simulink model "QSS_HEV"  (R2024a)
settings: Solver=VariableStepDiscrete  StartTime=0.0  StopTime=1220  RelTol=1e-3  EnableMultiTasking=on
undefined symbols (not defined in the file or in its folder): eta_EM_map, h, H_u, P_MGB_FTP75, PMGB_NEDC, rho_f, T_CE_max, T_EM_max, V_CE_map, w_CE_max, w_EM_row
libraries: qss_tb_library x7, simulink x2, dspindex x2, mpclib x1
settings Model: Creator=d_goerges  LastModifiedBy=apple
settings SolverCC: AlgebraicLoopSolver=TrustRegion
settings DataIOCC: LimitDataPoints=on  SaveFormat=Array  SignalLoggingSaveFormat=ModelDataLogs  ReturnWorkspaceOutputs=off
settings OptimizationCC: ExpressionDepthLimit=2147483647  LifeSpan=inf
settings DebuggingCC: UnderspecifiedInitializationDetection=Classic  MergeDetectMultiDrivingBlocksExec=none  SolverPrmCheckMsg=warning  FcnCallInpInsideContextMsg=warning  UnconnectedInputMsg=warning  UnconnectedOutputMsg=warning  UnconnectedLineMsg=warning  StateNameClashWarn=warning  SFUnexpectedBacktrackingDiag=warning  SFNoUnconditionalDefaultTransitionDiag=warning  SFExecutionAtInitializationDiag=none  ArithmeticOperatorsInVariantConditions=warning
settings HardwareCC: ProdBitPerPointer=32  ProdBitPerSizeT=32  ProdBitPerPtrDiffT=32  ProdLargestAtomicFloat=None  ProdIntDivRoundTo=Undefined  ProdEndianess=Unspecified  ProdWordSize=32  ProdHWDeviceType=32-bit Generic
settings ModelReferenceCC: PropagateSignalLabelsOutOfModel=off
settings SFSimCC: SimUseLocalCustomCode=off  CustomCodeUndefinedFunction=UseInterfaceOnly
settings RTWCC: RTWUseLocalCustomCode=off  GPUComputeCapability=3.5
settings CodeAppCC: StateflowObjectComments=on
settings GRTTargetCC: TargetLangStandard=C89/C90 (ANSI)  CombineOutputUpdateFcns=off  GRTInterface=on
settings ConfigComp: CovMetricSettings=dw  CovSaveCumulativeToWorkspaceVar=on  CovSaveSingleToWorkspaceVar=on  CovExternalEMLEnable=off

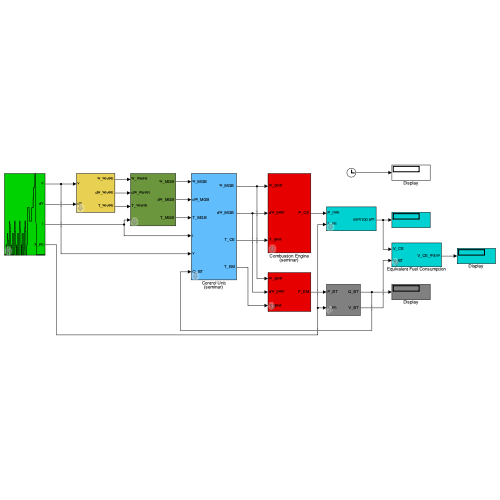
[thumbnail: Simulink's stored preview of the top-level diagram]
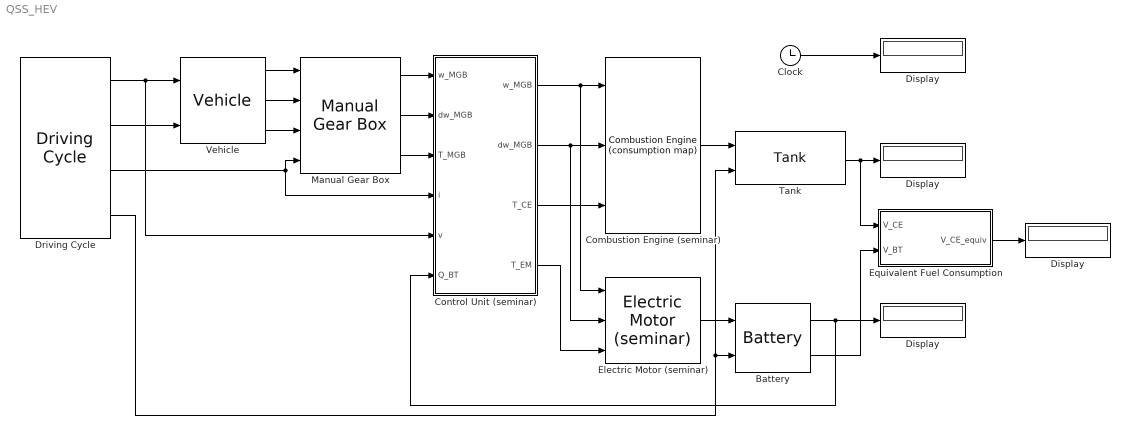
== system QSS_HEV ==
  "   Display   " : Display
  "  Display  " : Display
  " Display " : Display
  Battery : qss_tb_library/Energy Buffer/Battery  Tag=battery  I_0=10  Q_BT_IC_rel=50  t_ch=2
  Clock : Clock
  Combustion Engine (seminar) : qss_tb_library/Energy Converter/Combustion Engine (consumption map)  Tag=combustion engine  theta_CE=0.2  w_CE_idle=105  P_CE_idle=8000  P_aux=0  ENABLE_FUEL_CUTOFF=on  T_CE_cutoff=5  P_CE_cutoff=0
  Control Unit (seminar) : Subsystem  Tag=control unit  mask(Control Unit){}
      mask help:
      | This block gives the user the opportunity to design his/her own control unit.
      |
      | The user can define the inputs and outputs  by himself/herself.
      mask init:
      | %init_control_unit;
  Display : Display
  Driving Cycle : qss_tb_library/Driving Cycle/Driving Cycle  Tag=cycle  cyclenr=Europe: NEDC  stepsize=1  autostop=on
  Electric Motor (seminar) : qss_tb_library/Energy Converter/Electric Motor (seminar)  theta_EM=0.1  P_aux=0
  Equivalent Fuel Consumption : Subsystem  mask(Equivalent Fuel Consumption){eta_BT=0.9, eta_EM=0.8, eta_CE=0.25}
      mask prompts: eta_BT "Battery efficiency [-]"; eta_EM "Motor efficiency [-]"; eta_CE "Engine efficiency [-]"
      mask help:
      | This block computes the equivalent fuel consumption.
      |
      | Input:
      | =====
      | 	V_CE    Fuel consumption [l/100 km]
      | 	V_BT    Energy consumption [kWh/100 km]
      |
      | Output:
      | ======
      | 	V_CE_equiv	Equivalent fuel consumption [l/100 km]
      mask init:
      | init_equivalent_fuel_consumption;
  Manual Gear Box : qss_tb_library/Gear System/Manual Gear Box  Tag=transmission  i_1=3.27  i_2=1.92  i_3=1.26  i_4=0.88  i_5=0.7  i_diff=3.29  e_GT=0.98  P_GT0=100  w_wheel_min=1
  Tank : qss_tb_library/Energy Source/Tank  Tag=tank  fuel=Diesel  flag_cold_start=on
  Vehicle : qss_tb_library/Vehicle/Vehicle  Tag=vehicle  m_f=1115  mt2m_f=5  A_f=2.3  d_wheel=0.576  cw=0.31  mu=0.013
  wires:
  Tank/1 -> Display/1, Equivalent Fuel Consumption/1(V_CE)
  Driving Cycle/2 -> Vehicle/2
  Driving Cycle/1 -> Vehicle/1, Control Unit (seminar)/5(v)
  Vehicle/1 -> Manual Gear Box/1
  Vehicle/2 -> Manual Gear Box/2
  Vehicle/3 -> Manual Gear Box/3
  Manual Gear Box/1 -> Control Unit (seminar)/1(w_MGB)
  Manual Gear Box/2 -> Control Unit (seminar)/2(dw_MGB)
  Manual Gear Box/3 -> Control Unit (seminar)/3(T_MGB)
  Control Unit (seminar)/1(" w_MGB ") -> Combustion Engine (seminar)/1, Electric Motor (seminar)/1
  Control Unit (seminar)/2(" dw_MGB ") -> Combustion Engine (seminar)/2, Electric Motor (seminar)/2
  Control Unit (seminar)/3(T_CE) -> Combustion Engine (seminar)/3
  Control Unit (seminar)/4(T_EM) -> Electric Motor (seminar)/3
  Combustion Engine (seminar)/1 -> Tank/1
  Electric Motor (seminar)/1 -> Battery/1
  Driving Cycle/4 -> Battery/2, Tank/2
  Battery/1 -> "  Display  "/1, Control Unit (seminar)/6(Q_BT)
  Driving Cycle/3 -> Manual Gear Box/4, Control Unit (seminar)/4(i)
  Battery/2 -> Equivalent Fuel Consumption/2(V_BT)
  Clock/1 -> " Display "/1
  Equivalent Fuel Consumption/1(V_CE_equiv) -> "   Display   "/1

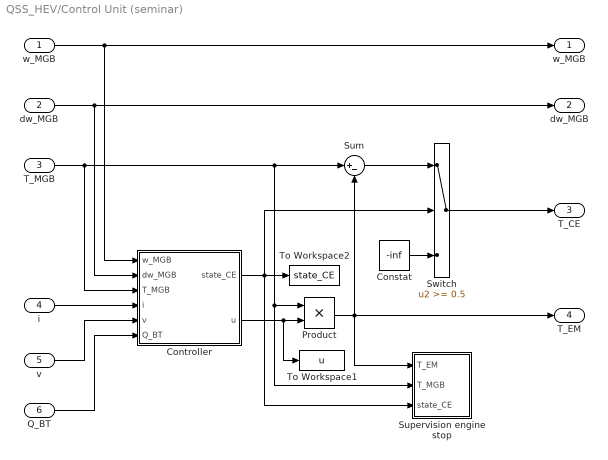
== system QSS_HEV/Control Unit (seminar) ==
  w_MGB : Inport
  dw_MGB : Inport  Port=2
  T_MGB : Inport  Port=3
  i : Inport  Port=4
  v : Inport  Port=5
  Q_BT : Inport  Port=6
  Constat : Constant  Value=-inf
  Controller : Subsystem  TreatAsAtomicUnit=on
  Product : Product  RndMeth=Zero
  Sum : Sum  Inputs=|+-
  Supervision engine stop : Subsystem
  Switch : Switch  Threshold=0.5  SaturateOnIntegerOverflow=off  InputSameDT=off
  To Workspace1 : ToWorkspace  VariableName=u  SampleTime=-1
  To Workspace2 : ToWorkspace  VariableName=state_CE  SampleTime=-1
  " w_MGB " : Outport  InitialOutput=0
  " dw_MGB " : Outport  Port=2  InitialOutput=0
  T_CE : Outport  Port=3  InitialOutput=0
  T_EM : Outport  Port=4  InitialOutput=0
  wires:
  dw_MGB/1 -> Controller/2(dw_MGB), " dw_MGB "/1
  w_MGB/1 -> Controller/1(w_MGB), " w_MGB "/1
  T_MGB/1 -> Controller/3(T_MGB), Sum/1, Product/1, Supervision engine stop/2(T_MGB)
  Product/1 -> Sum/2, T_EM/1, Supervision engine stop/1(T_EM)
  Controller/2(u) -> To Workspace1/1, Product/2
  i/1 -> Controller/4(i)
  Controller/1(state_CE) -> Switch/2, To Workspace2/1, Supervision engine stop/3(state_CE)
  Sum/1 -> Switch/1
  Switch/1 -> T_CE/1
  Constat/1 -> Switch/3
  v/1 -> Controller/5(v)
  Q_BT/1 -> Controller/6(Q_BT)

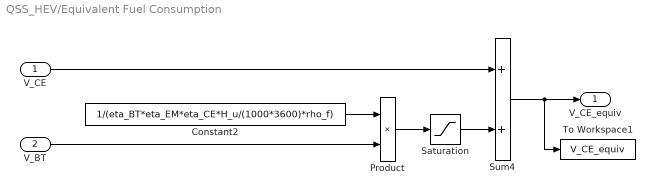
== system QSS_HEV/Equivalent Fuel Consumption ==
  V_CE : Inport
  V_BT : Inport  Port=2
  Constant2 : Constant  Value=1/(eta_BT*eta_EM*eta_CE*H_u/(1000*3600)*rho_f)
  Product : Product  RndMeth=Zero
  Saturation : Saturate  UpperLimit=inf  LowerLimit=0
  Sum4 : Sum  InputSameDT=on  SaturateOnIntegerOverflow=on  OutDataTypeStr=Inherit: Same as first input
  To Workspace1 : ToWorkspace  VariableName=V_CE_equiv  SampleTime=-1
  V_CE_equiv : Outport
  wires:
  Product/1 -> Saturation/1
  V_BT/1 -> Product/2
  Constant2/1 -> Product/1
  Sum4/1 -> To Workspace1/1, V_CE_equiv/1
  V_CE/1 -> Sum4/1
  Saturation/1 -> Sum4/2

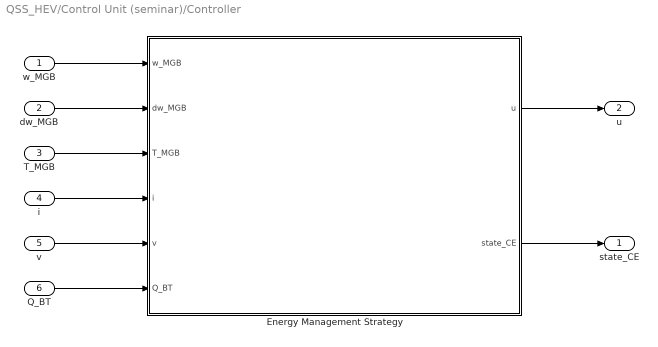
== system QSS_HEV/Control Unit (seminar)/Controller ==
  w_MGB : Inport
  dw_MGB : Inport  Port=2
  T_MGB : Inport  Port=3
  i : Inport  Port=4
  v : Inport  Port=5
  Q_BT : Inport  Port=6
  Energy Management Strategy : Subsystem
  state_CE : Outport  InitialOutput=0
  u : Outport  Port=2  InitialOutput=0
  wires:
  Energy Management Strategy/2(state_CE) -> state_CE/1
  Energy Management Strategy/1(u) -> u/1
  w_MGB/1 -> Energy Management Strategy/1(w_MGB)
  dw_MGB/1 -> Energy Management Strategy/2(dw_MGB)
  T_MGB/1 -> Energy Management Strategy/3(T_MGB)
  i/1 -> Energy Management Strategy/4(i)
  v/1 -> Energy Management Strategy/5(v)
  Q_BT/1 -> Energy Management Strategy/6(Q_BT)

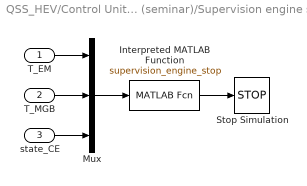
== system QSS_HEV/Control Unit (seminar)/Supervision engine stop ==
  T_EM : Inport
  T_MGB : Inport  Port=2
  state_CE : Inport  Port=3
  Interpreted MATLAB Function : MATLABFcn  MATLABFcn=supervision_engine_stop
  Mux : Mux  Inputs=3
  Stop Simulation : Stop
  wires:
  T_MGB/1 -> Mux/2
  T_EM/1 -> Mux/1
  state_CE/1 -> Mux/3
  Mux/1 -> Interpreted MATLAB Function/1
  Interpreted MATLAB Function/1 -> Stop Simulation/1

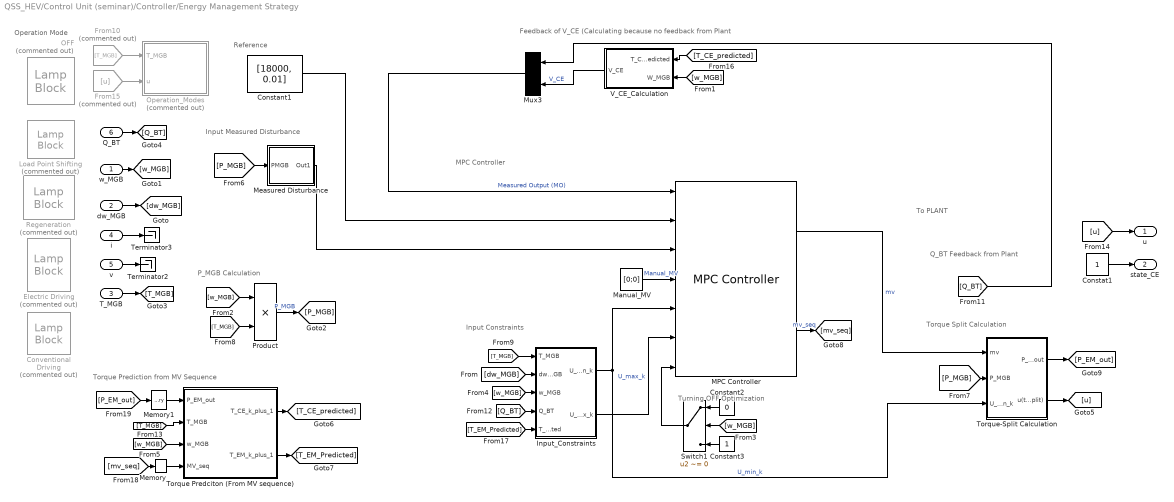
== system QSS_HEV/Control Unit (seminar)/Controller/Energy Management Strategy ==
  note: Q_BT Feedback from Plant
  note: Torque Split Calculation
  note: Input Constraints
  note: To PLANT
  note: MPC Controller
  note: Feedback of V_CE (Calculating because no feedback from Plant
  note: Turning OFF Optimization
  note: Input Measured Disturbance
  note: Reference
  note: Torque Prediction from MV Sequence
  note: P_MGB Calculation
  note: Operation Mode
  w_MGB : Inport
  dw_MGB : Inport  Port=2
  T_MGB : Inport  Port=3
  i : Inport  Port=4
  v : Inport  Port=5
  Q_BT : Inport  Port=6
  Constant1 : Constant  Value=[18000, 0.01]  VectorParams1D=off
  Constant2 : Constant  Value=0
  Constant3 : Constant
  Constat1 : Constant
  Conventional Driving : LampBlock  Commented=on  LabelPosition=Hide
  Electric Driving : LampBlock  Commented=on  LabelPosition=Hide
  From10 : From  Commented=on  GotoTag=T_MGB
  From15 : From  Commented=on  GotoTag=u
  Input_Constraints : Subsystem
  "Load Point Shifting " : LampBlock  Commented=on  LabelPosition=Hide
  MPC Controller : mpclib/MPC Controller  SCDEnableBlockLinearizationSpecification=on  mpcobj=mpc_object  is_multiple=0  enable_value=0  return_u0=off  updateMPCinCallerWorkspace=on  md_inport=on  mv_inport=on  uref_inport=off  return_cost=off  return_mvseq=on  return_qpstatus=off  return_xseq=off  return_state=off  return_ovseq=off  state_inport=off  umin_inport=on  umax_inport=on  ymin_inport=off  ymax_inport=off  cc_inport=off  ywt_inport=off  uwt_inport=off  duwt_inport=off  rhoeps_inport=off  pm_inport=off  MaximumP=10  HorizonChoice=FixedHorizon  n_ts=1  n_p=11  n_mv=2  n_md=1  n_ud=0  n_mo=2  n_uo=0  BlockDataType=double  SampleTimeInherited=off  switch_inport=on
  Manual_MV : Constant  Value=[0;0]  VectorParams1D=off
  Measured Disturbance : Subsystem
  Memory : Memory
  Memory1 : Memory
  Mux3 : Mux  Inputs=2
  OFF : LampBlock  Commented=on  LabelPosition=Hide
  Operation_Modes : Stateflow chart  Commented=on  TreatAsAtomicUnit=on
  Product : Product  OutDataTypeStr=double
  Regeneration : LampBlock  Commented=on  LabelPosition=Hide
  Switch1 : Switch  Criteria=u2 ~= 0  SaturateOnIntegerOverflow=off  InputSameDT=off
  Terminator2 : Terminator
  Terminator3 : Terminator
  Torque Predciton (From MV sequence) : MATLAB Function  TreatAsAtomicUnit=on
  Torque-Split Calculation : Subsystem
  V_CE_Calculation : Subsystem
  u : Outport
  state_CE : Outport  Port=2
  wires:
  T_MGB/1 -> [T_MGB]
  Constat1/1 -> state_CE/1
  [Q_BT] -> Input_Constraints/4(Q_BT)
  Constant1/1 -> MPC Controller/2
  [T_MGB] -> Torque Predciton (From MV sequence)/2(T_MGB)
  Torque Predciton (From MV sequence)/1(T_CE_k_plus_1) -> [T_CE_predicted]
  dw_MGB/1 -> [dw_MGB]
  i/1 -> Terminator3/1
  Switch1/1 -> MPC Controller/7
  [T_MGB] -> Product/2
  [w_MGB] -> Switch1/2
  [P_MGB] -> Measured Disturbance/1(PMGB)
  Measured Disturbance/1(Out1) -> MPC Controller/3
  [T_CE_predicted] -> V_CE_Calculation/1(T_CE_k_predicted)
  [Q_BT] -> Mux3/1
  [T_MGB] -> Input_Constraints/1(T_MGB)
  V_CE_Calculation/1(V_CE) -> Mux3/2  "V_CE"
  Q_BT/1 -> [Q_BT]
  From10/1 -> Operation_Modes/1(T_MGB)
  [w_MGB] -> Torque Predciton (From MV sequence)/3(w_MGB)
  [w_MGB] -> V_CE_Calculation/2(W_MGB)
  [w_MGB] -> Product/1
  [w_MGB] -> Input_Constraints/3(w_MGB)
  Product/1 -> [P_MGB]  "P_MGB"
  v/1 -> Terminator2/1
  [u] -> u/1
  w_MGB/1 -> [w_MGB]
  Input_Constraints/2(U_max_k) -> MPC Controller/6  "U_max_k"
  Input_Constraints/1(U_min_k) -> Torque-Split Calculation/3(U_min_k), MPC Controller/5  "U_min_k"
  Mux3/1 -> MPC Controller/1  "Measured Output (MO)"
  Constant2/1 -> Switch1/1
  From15/1 -> Operation_Modes/2(u)
  Constant3/1 -> Switch1/3
  [dw_MGB] -> Input_Constraints/2(dw_MGB)
  Manual_MV/1 -> MPC Controller/4  "Manual_MV"
  Memory/1 -> Torque Predciton (From MV sequence)/4(MV_seq)
  MPC Controller/1 -> Torque-Split Calculation/1(mv)  "mv"
  [P_MGB] -> Torque-Split Calculation/2(P_MGB)
  Torque-Split Calculation/1(P_EM_out) -> [P_EM_out]
  Torque-Split Calculation/2(u(torque split)) -> [u]
  [T_EM_Predicted] -> Input_Constraints/5(T_EM_Predicted)
  Torque Predciton (From MV sequence)/2(T_EM_k_plus_1) -> [T_EM_Predicted]
  MPC Controller/2 -> [mv_seq]  "mv_seq"
  [mv_seq] -> Memory/1
  [P_EM_out] -> Memory1/1
  Memory1/1 -> Torque Predciton (From MV sequence)/1(P_EM_out)

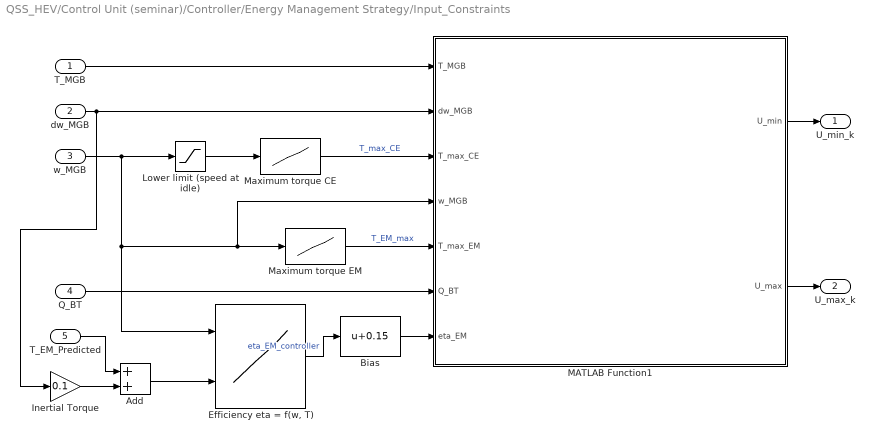
== system QSS_HEV/Control Unit (seminar)/Controller/Energy Management Strategy/Input_Constraints ==
  T_MGB : Inport
  dw_MGB : Inport  Port=2
  w_MGB : Inport  Port=3
  Q_BT : Inport  Port=4
  T_EM_Predicted : Inport  Port=5
  Add : Sum
  Bias : Bias  Bias=0.15  SaturateOnIntegerOverflow=off
  "Efficiency eta = f(w, T)" : Lookup2D  RowIndex=w_EM_row  ColumnIndex=T_EM_col  Table=eta_EM_map  InputSameDT=off
  Inertial Torque : Gain  Gain=0.1
  Lower limit (speed at idle) : Saturate  UpperLimit=inf  LowerLimit=105
  MATLAB Function1 : MATLAB Function  TreatAsAtomicUnit=on
  Maximum torque CE : Lookup  InputValues=w_CE_max  Table=T_CE_max
  Maximum torque EM : Lookup  InputValues=w_EM_row  Table=T_EM_max
  U_min_k : Outport
  U_max_k : Outport  Port=2
  wires:
  w_MGB/1 -> "Efficiency eta = f(w, T)"/1, MATLAB Function1/4(w_MGB), Maximum torque EM/1, Lower limit (speed at idle)/1
  Maximum torque CE/1 -> MATLAB Function1/3(T_max_CE)  "T_max_CE"
  Maximum torque EM/1 -> MATLAB Function1/5(T_max_EM)  "T_EM_max"
  Lower limit (speed at idle)/1 -> Maximum torque CE/1
  dw_MGB/1 -> Inertial Torque/1, MATLAB Function1/2(dw_MGB)
  T_MGB/1 -> MATLAB Function1/1(T_MGB)
  MATLAB Function1/1(U_min) -> U_min_k/1
  MATLAB Function1/2(U_max) -> U_max_k/1
  Q_BT/1 -> MATLAB Function1/6(Q_BT)
  "Efficiency eta = f(w, T)"/1 -> Bias/1  "eta_EM_controller"
  T_EM_Predicted/1 -> Add/1
  Bias/1 -> MATLAB Function1/7(eta_EM)
  Inertial Torque/1 -> Add/2
  Add/1 -> "Efficiency eta = f(w, T)"/2

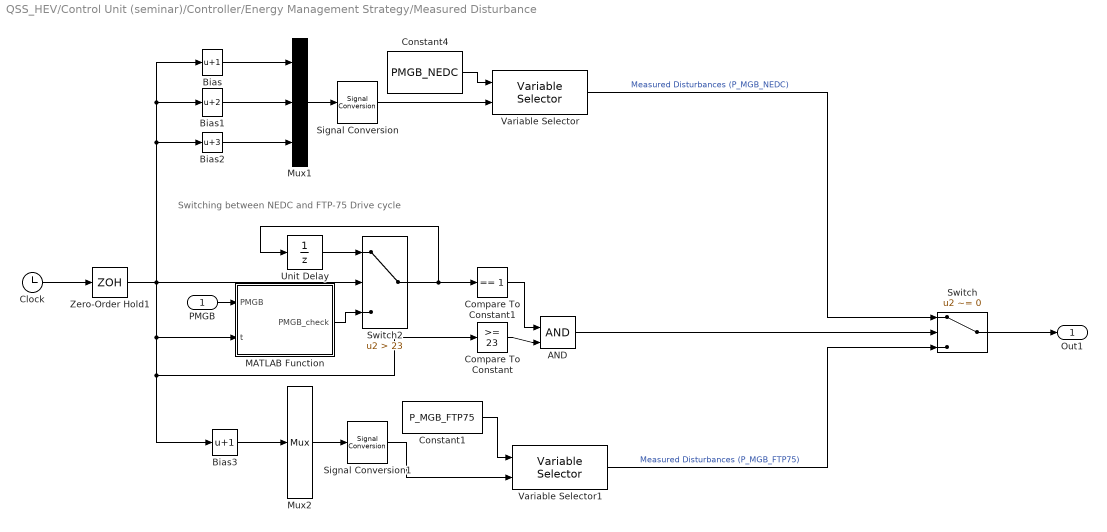
== system QSS_HEV/Control Unit (seminar)/Controller/Energy Management Strategy/Measured Disturbance ==
  note: Switching between NEDC and FTP-75 Drive cycle
  PMGB : Inport
  AND : Logic  IconShape=distinctive  AllPortsSameDT=off  OutDataTypeStr=boolean
  Bias : Bias  Bias=1  SaturateOnIntegerOverflow=off
  Bias1 : Bias  Bias=2  SaturateOnIntegerOverflow=off
  Bias2 : Bias  Bias=3  SaturateOnIntegerOverflow=off
  Bias3 : Bias  Bias=1  SaturateOnIntegerOverflow=off
  Clock : Clock
  Compare To Constant : simulink/Logic and Bit Operations/Compare To Constant  relop=>=  const=23  OutDataTypeStr=boolean
  Compare To Constant1 : simulink/Logic and Bit Operations/Compare To Constant  relop===  const=1  OutDataTypeStr=boolean
  Constant1 : Constant  Value=P_MGB_FTP75
  Constant4 : Constant  Value=PMGB_NEDC
  MATLAB Function : MATLAB Function  TreatAsAtomicUnit=on
  Mux1 : Mux  Inputs=3
  Mux2 : Mux  Inputs=1
  Signal Conversion : SignalConversion  OverrideOpt=off
  Signal Conversion1 : SignalConversion  OverrideOpt=off
  Switch : Switch  Criteria=u2 ~= 0  SaturateOnIntegerOverflow=off  InputSameDT=off
  Switch2 : Switch  Criteria=u2 > Threshold  Threshold=23  SaturateOnIntegerOverflow=off  InputSameDT=off
  Unit Delay : UnitDelay  SampleTime=-1  HasFrameUpgradeWarning=on
  Variable Selector : dspindex/Variable Selector  NumInputs=1  rowsOrCols=Rows  IdxMode=Variable  Elements=[1 3]  ZerOneIdxMode=One-based  errmode=Clip Index  FillMode=on  FillValues=0
  Variable Selector1 : dspindex/Variable Selector  NumInputs=1  rowsOrCols=Rows  IdxMode=Variable  Elements=[1 3]  ZerOneIdxMode=One-based  errmode=Clip Index  FillMode=on  FillValues=0
  Zero-Order Hold1 : ZeroOrderHold  SampleTime=-1
  Out1 : Outport
  wires:
  Bias/1 -> Mux1/1
  Mux1/1 -> Signal Conversion/1
  Clock/1 -> Zero-Order Hold1/1
  Variable Selector/1 -> Switch/1  "Measured Disturbances (P_MGB_NEDC)"
  Bias1/1 -> Mux1/2
  Signal Conversion/1 -> Variable Selector/2
  Constant4/1 -> Variable Selector/1
  Compare To Constant/1 -> AND/2
  AND/1 -> Switch/2
  Switch/1 -> Out1/1
  PMGB/1 -> MATLAB Function/1(PMGB)
  Bias2/1 -> Mux1/3
  MATLAB Function/1(PMGB_check) -> Switch2/3
  Switch2/1 -> Compare To Constant1/1, Unit Delay/1
  Unit Delay/1 -> Switch2/1
  Compare To Constant1/1 -> AND/1
  Bias3/1 -> Mux2/1
  Mux2/1 -> Signal Conversion1/1
  Constant1/1 -> Variable Selector1/1
  Zero-Order Hold1/1 -> Bias3/1, Compare To Constant/1, MATLAB Function/2(t), Bias2/1, Bias1/1, Bias/1, Switch2/2
  Variable Selector1/1 -> Switch/3  "Measured Disturbances (P_MGB_FTP75)"
  Signal Conversion1/1 -> Variable Selector1/2

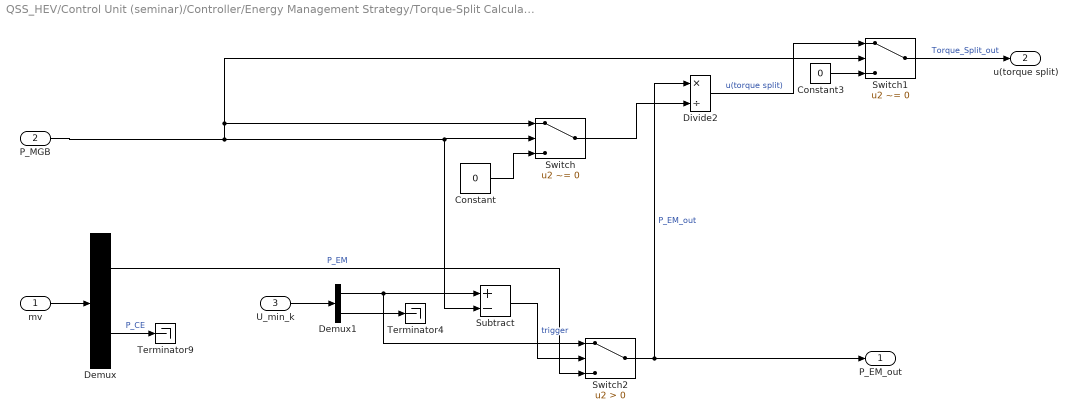
== system QSS_HEV/Control Unit (seminar)/Controller/Energy Management Strategy/Torque-Split Calculation ==
  mv : Inport
  P_MGB : Inport  Port=2
  U_min_k : Inport  Port=3
  Constant : Constant  Value=0
  Constant3 : Constant  Value=0
  Demux : Demux  Outputs=2
  Demux1 : Demux  Outputs=2
  Divide2 : Product  Inputs=*/
  Subtract : Sum  Inputs=+-
  Switch : Switch  Criteria=u2 ~= 0  SaturateOnIntegerOverflow=off  InputSameDT=off
  Switch1 : Switch  Criteria=u2 ~= 0  SaturateOnIntegerOverflow=off  InputSameDT=off
  Switch2 : Switch  Criteria=u2 > Threshold  SaturateOnIntegerOverflow=off  InputSameDT=off
  Terminator4 : Terminator
  Terminator9 : Terminator
  P_EM_out : Outport
  u(torque split) : Outport  Port=2
  wires:
  mv/1 -> Demux/1
  U_min_k/1 -> Demux1/1
  Demux1/2 -> Terminator4/1
  Demux/1 -> Switch2/3  "P_EM"
  Demux/2 -> Terminator9/1  "P_CE"
  Demux1/1 -> Switch2/1, Subtract/1
  P_MGB/1 -> Subtract/2, Switch/2, Switch/1, Switch1/2
  Switch2/1 -> P_EM_out/1, Divide2/1  "P_EM_out"
  Subtract/1 -> Switch2/2  "trigger"
  Switch1/1 -> u(torque split)/1  "Torque_Split_out"
  Divide2/1 -> Switch1/1  "u(torque split)"
  Constant3/1 -> Switch1/3
  Switch/1 -> Divide2/2
  Constant/1 -> Switch/3

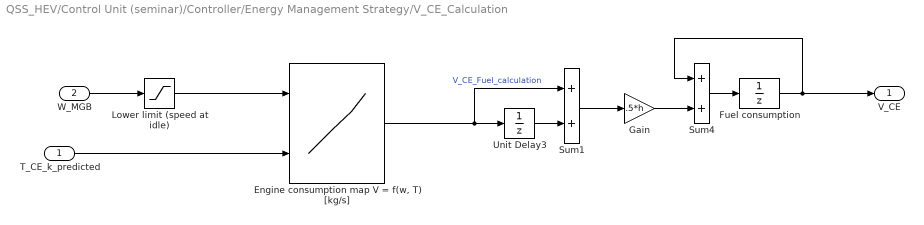
== system QSS_HEV/Control Unit (seminar)/Controller/Energy Management Strategy/V_CE_Calculation ==
  T_CE_k_predicted : Inport
  W_MGB : Inport  Port=2
  "Engine consumption map V = f(w, T) [kg/s]" : Lookup2D  RowIndex=w_CE_row  ColumnIndex=T_CE_col  Table=V_CE_map  SaturateOnIntegerOverflow=off  InputSameDT=off
  Fuel consumption : UnitDelay  SampleTime=h  HasFrameUpgradeWarning=on
  Gain : Gain  Gain=.5*h
  Lower limit (speed at idle) : Saturate  UpperLimit=inf  LowerLimit=105
  Sum1 : Sum  InputSameDT=on  SaturateOnIntegerOverflow=on  OutDataTypeStr=Inherit: Same as first input
  Sum4 : Sum  InputSameDT=on  SaturateOnIntegerOverflow=on  OutDataTypeStr=Inherit: Same as first input
  Unit Delay3 : UnitDelay  SampleTime=h  HasFrameUpgradeWarning=on
  V_CE : Outport
  wires:
  T_CE_k_predicted/1 -> "Engine consumption map V = f(w, T) [kg/s]"/2
  W_MGB/1 -> Lower limit (speed at idle)/1
  Sum4/1 -> Fuel consumption/1
  Sum1/1 -> Gain/1
  "Engine consumption map V = f(w, T) [kg/s]"/1 -> Sum1/1, Unit Delay3/1  "V_CE_Fuel_calculation"
  Gain/1 -> Sum4/2
  Unit Delay3/1 -> Sum1/2
  Lower limit (speed at idle)/1 -> "Engine consumption map V = f(w, T) [kg/s]"/1
  Fuel consumption/1 -> Sum4/1, V_CE/1

== matlab function QSS_HEV/Control Unit (seminar)/Controller/Energy Management Strategy/Torque Predciton (From MV sequence) ==
  data: P_EM_out input; T_MGB input; w_MGB input; MV_seq input; T_CE_k_plus_1 output; T_EM_k_plus_1 output
function [T_CE_k_plus_1,T_EM_k_plus_1] = T_Prediction(P_EM_out,T_MGB, w_MGB, MV_seq)
T_EM_k_plus_1 = 0;
PCE_K_plus_1 = MV_seq(2,2);
PEM_K_plus_1 = MV_seq(2,1);
if w_MGB > 105
    T_CE_k_plus_1 = PCE_K_plus_1/w_MGB;
else
    T_CE_k_plus_1 = 0;
end
if T_MGB >=0
    if w_MGB == 0
        T_EM_k_plus_1 = 0;
    else 
        T_EM_k_plus_1 = PEM_K_plus_1/w_MGB;
    end
else
    if w_MGB ~= 0
        T_EM_k_plus_1 = P_EM_out/w_MGB;
    else
    end

end

end

== matlab function QSS_HEV/Control Unit (seminar)/Controller/Energy Management Strategy/Input_Constraints/MATLAB Function1 ==
  data: T_MGB input; dw_MGB input; T_max_CE input; w_MGB input; U_min output; T_max_EM input; U_max output; Q_BT input; eta_EM input
function [U_min,U_max] = Input_Constraints(T_MGB, dw_MGB, T_max_CE, w_MGB, T_max_EM, Q_BT, eta_EM)

delta_t = 1;
delta_p = delta_t * w_MGB;
theta_CE = 0.2;
theta_EM = 0.1;

% Battery Parameters
c_BT_E1     =  39;                          % Minimum battery voltage for discharging (13 cells, 3 V/cell, seminar)                 [V]
c_BT_E2     =  0.013;					    % Minimum battery resistance for discharging (13 cells, 1 mOhm/cell, seminar)           [Ohm]
c_BT_E3     =  15.6;					    % Maximum battery voltage variation for discharging (13 cells, 1.2 V/cell, seminar)     [V]
c_BT_E4     =  0;							% Minimum battery resistance variation for discharging (13 cells, 0 mOhm/cell, seminar) [Ohm]
c_BT_L1     =  c_BT_E1;                     % c_BT_L1 = c_BT_EL1 for continuity reasons
c_BT_L2     =  0.013;					    % Minimum battery resistance for charging (13 cells, 1 mOhm/cell, seminar)              [V]
c_BT_L3     =  c_BT_E3;                     % c_BT_L3 = c_BT_EL3 for continuity reasons
c_BT_L4     =  0.00;                        % Minimum battery resistance variation for charging (13 cells, 0 mOhm/cell, seminar)    [Ohm]

I_0 = 10;

Q_bt0      = I_0 * 3600;					% Discharge current in 1 h              [C]
I_bt_max    = (60/2)*I_0;			    	% Maximum charge/discharge current      [A]

%%
% During discharging 
AE1_discharge = (c_BT_E3 * (Q_BT/Q_bt0)) + c_BT_E1;
AE2_discharge = (c_BT_E4) * (Q_BT/Q_bt0) + c_BT_E2;
P_BT_discharge = I_bt_max^2 * ((AE1_discharge/I_bt_max) - (AE2_discharge/I_0));

% During charging
AE1_charge = (c_BT_L3 * (Q_BT/Q_bt0)) + c_BT_L1;
AE2_charge = (c_BT_L4) * (Q_BT/Q_bt0) + c_BT_L2;
P_BT_charge = -(I_bt_max^2 * ((AE1_charge/I_bt_max) - (AE2_charge/I_0)));

%% CE Constraints
T_CE_inertia = abs(theta_CE* dw_MGB);       % Inertial Torque of CE
% Upper Limit of P_CE
T_CE_upper = T_max_CE-delta_t -T_CE_inertia;
P_CE_max = T_CE_upper*w_MGB;

% Lower Limit of P_CE 
P_CE_min = 0;
  

%% EM Constraints

T_EM_inertia = abs(theta_EM* dw_MGB);
% Upper Limit of P_EM

    if w_MGB > 0
        T_EM_upper = T_max_EM - T_EM_inertia - delta_t;
    else
        T_EM_upper = T_max_EM -T_EM_inertia;                % delta is not include because at w_MGB =0, T_EM should be 0
    end
    
P_EM_lim_max = T_EM_upper * w_MGB;
P_em_cur_max = P_BT_discharge/eta_EM - (T_EM_inertia * w_MGB);
P_EM_max = min(P_EM_lim_max,P_em_cur_max-delta_p);

% Lower Limit of P_EM
if T_MGB >=0
    T_EM_lower = -T_EM_upper;
else
    T_EM_lower = max(T_MGB+delta_t, -T_EM_upper);
end

P_EM_lim_min = T_EM_lower * w_MGB;

P_em_cur_min = P_BT_charge/eta_EM -(T_EM_inertia*w_MGB);
P_EM_min = max(P_EM_lim_min,P_em_cur_min+delta_p);

U_min = [P_EM_min;P_CE_min];
U_max = [P_EM_max;P_CE_max];

== matlab function QSS_HEV/Control Unit (seminar)/Controller/Energy Management Strategy/Measured Disturbance/MATLAB Function ==
  data: PMGB input; PMGB_check output; t input
function PMGB_check = fcn(PMGB,t) 
PMGB_check = zeros(1);
if t == 23 && PMGB == 0
     PMGB_check = 1;
elseif t == 23 && PMGB ~= 0 
     PMGB_check = 2;
end

== stateflow chart QSS_HEV/Control Unit (seminar)/Controller/Energy Management Strategy/Operation_Modes ==
  state Conventional_Driving
    entry:
    OFF_States = 0;
    LPS = 0;
    ED=0;
    REG=0;
    CD=1;
  state Regeneration
    entry:
    OFF_States = 0;
    LPS = 0;
    ED=0;
    REG=1;
    CD=0;
  state Load_Point_Shifting
    entry:
    OFF_States = 0;
    LPS = 1;
    ED=0;
    REG=0;
    CD=0;
  state OFF
    entry:
    OFF_States = 1;
    LPS = 0;
    ED=0;
    REG=0;
    CD=0;
    OFF -> OFF [order 1]
  state Electric_Driving
    entry:
    OFF_States = 0;
    LPS = 0;
    ED=1;
    REG=0;
    CD=0;
  Electric_Driving -> Conventional_Driving [order 4] : [T_MGB > 0 & u == 0]
  Conventional_Driving -> Electric_Driving [order 4] : [[T_MGB > 0 & u == 1]]
  Load_Point_Shifting -> Conventional_Driving [order 4] : [T_MGB > 0 & u == 0]
  Regeneration -> Conventional_Driving [order 4] : [T_MGB > 0 & u == 0]
  Conventional_Driving -> Load_Point_Shifting [order 1] : [[(T_MGB >0 & 0 < u & u < 1) | (T_MGB > 0 & u < 0)]]
  Conventional_Driving -> Regeneration [order 2] : [(T_MGB <0 & u == 1) | (T_MGB < 0 & 0 <= u & u < 1)]
  Conventional_Driving -> OFF [order 3] : [[T_MGB == 0 & u == 0]]
  OFF -> Conventional_Driving [order 4] : [T_MGB > 0 & u == 0]
  Load_Point_Shifting -> Regeneration [order 2] : [(T_MGB <0 & u == 1) | (T_MGB < 0 & 0 <= u & u < 1)]
  Regeneration -> Load_Point_Shifting [order 1] : [[(T_MGB >0 & 0 < u & u < 1) | (T_MGB > 0 & u < 0)]]
  (default) -> OFF
  Load_Point_Shifting -> OFF [order 3] : [T_MGB == 0 & u == 0]
  Regeneration -> OFF [order 3] : [T_MGB == 0 & u == 0]
  OFF -> Load_Point_Shifting [order 1] : [[(T_MGB >0 & 0 < u & u < 1) | (T_MGB > 0 & u < 0)]]
  OFF -> Regeneration [order 2] : [[(T_MGB <0 & u == 1) | (T_MGB < 0 & 0 <= u & u < 1)]]
  Electric_Driving -> OFF [order 3] : [T_MGB == 0 & u == 0]
  OFF -> Electric_Driving [order 3] : [[T_MGB > 0 & u == 1]]
  Electric_Driving -> Load_Point_Shifting [order 2] : [(T_MGB >0 & 0 < u & u < 1) | (T_MGB > 0 & u < 0)]
  Load_Point_Shifting -> Electric_Driving [order 1] : [T_MGB > 0 & u== 1]
  Electric_Driving -> Regeneration [order 1] : [(T_MGB <0 & u == 1) | (T_MGB < 0 & 0 <= u & u < 1)]
  Regeneration -> Electric_Driving [order 2] : [T_MGB > 0 & u == 1]
  data: T_MGB input; u input; OFF_States local; LPS local; ED local; REG local; CD local
